simulink model "CascadePID_sim_v2"  (R2024b)
settings: Solver=ode1  StartTime=0.0  StopTime=1  FixedStep=0.005  RelTol=1e-3
undefined symbols (not defined in the file or in its folder): A, b_moment, g, k_thrust, l, M, m, T
libraries: simulink_extras x7, slpidlib x6
settings Model: Creator=Admin  LastModifiedBy=Admin

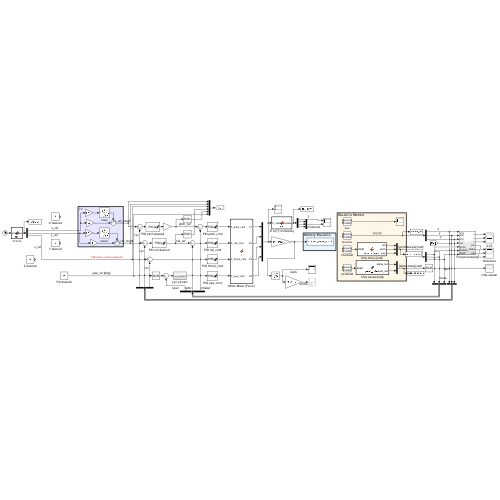
[thumbnail: Simulink's stored preview of the top-level diagram]
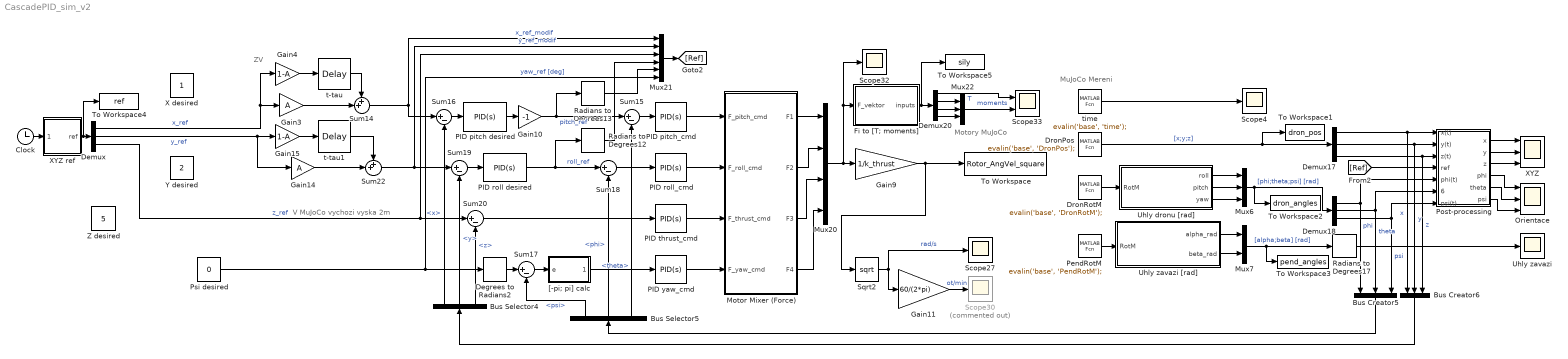
== system CascadePID_sim_v2 ==
  note: Motory MuJoCo
  note: V MuJoCo vychozi vyska 2m
  note: MuJoCo Mereni
  note: ZV
  Bus Creator5 : BusCreator  Inputs=3
  Bus Creator6 : BusCreator  Inputs=3
  Bus Selector4 : BusSelector  OutputSignals=x,y,z
  Bus Selector5 : BusSelector  OutputSignals=psi,phi,theta
  Clock : Clock
  Degrees to Radians2 : simulink_extras/Transformations/Degrees to Radians
  Demux : Demux  Outputs=3
  Demux17 : Demux  Outputs=3
  Demux18 : Demux  Outputs=3
  Demux20 : Demux
  DronPos : MATLABFcn  MATLABFcn=evalin('base', 'DronPos');  OutputDimensions=[3,1]  Output1D=off
  DronRotM : MATLABFcn  MATLABFcn=evalin('base', 'DronRotM');  OutputDimensions=[3,3]  Output1D=off
  Fi to [T; moments] : MATLAB Function  TreatAsAtomicUnit=on
  Gain10 : Gain  Gain=-1
  Gain11 : Gain  Gain=60/(2*pi)
  Gain14 : Gain  Gain=A
  Gain15 : Gain  Gain=1-A
  Gain3 : Gain  Gain=A
  Gain4 : Gain  Gain=1-A
  Gain9 : Gain  Gain=1/k_thrust
  Motor Mixer (Force) : MATLAB Function  TreatAsAtomicUnit=on
  Mux20 : Mux
  Mux21 : Mux  Inputs=6
  Mux22 : Mux  Inputs=3
  Mux6 : Mux  Inputs=3
  Mux7 : Mux  Inputs=2
  Orientace : Scope  NumInputPorts=3
  PID pitch desired : slpidlib/PID Controller  Controller=PID  Form=Parallel  TimeDomain=Continuous-time  UseExternalTs=off  SampleTime=-1  IntegratorMethod=Forward Euler  FilterMethod=Forward Euler  ControllerParametersSource=internal  P=-0.0958604126455568  I=-0.00355407713511052  UseKiTs=off  D=-0.176236133491369  UseExternalDerivativeSource=off  N=18.7292151918558  UseFilter=on  TunerSelectOption=Transfer Function Based (PID Tuner App)  InitialConditionSource=internal  InitialConditionForIntegrator=0  InitialConditionForFilter=0  DifferentiatorICPrevScaledInput=0  ExternalReset=none  TrackingMode=off  Kt=1  LimitOutput=on  SatLimitsSource=internal  UpperSaturationLimit=45*pi/180  LowerSaturationLimit=-45*pi/180  LinearizeAsGain=on  AntiWindupMode=clamping  Kb=1  LimitIntegrator=off  UpperIntegratorSaturationLimit=inf  LowerIntegratorSaturationLimit=-inf  POutMin=[]  POutMax=[]  IOutMin=[]  IOutMax=[]  DOutMin=[]  DOutMax=[]  NOutMin=[]  NOutMax=[]  SumOutMin=[]  SumOutMax=[]  SaturationOutMin=[]  SaturationOutMax=[]  PParamMin=[]  PParamMax=[]  IParamMin=[]  IParamMax=[]  DParamMin=[]  DParamMax=[]  NParamMin=[]  NParamMax=[]  KbParamMin=[]  KbParamMax=[]  KtParamMin=[]  KtParamMax=[]  KbOutMin=[]  KbOutMax=[]  KtOutMin=[]  KtOutMax=[]  IntegratorOutMin=[]  IntegratorOutMax=[]  FilterOutMin=[]  FilterOutMax=[]  SumI1OutMin=[]  SumI1OutMax=[]  SumI2OutMin=[]  SumI2OutMax=[]  SumI3OutMin=[]  SumI3OutMax=[]  SumI4OutMin=[]  SumI4OutMax=[]  SumDOutMin=[]  SumDOutMax=[]  DifferentiatorOutMin=[]  DifferentiatorOutMax=[]  FilterDiffOutCoefMin=[]  FilterDiffOutCoefMax=[]  ReciprocalOutMin=[]  ReciprocalOutMax=[]  SumDenOutMin=[]  SumDenOutMax=[]  SumNumOutMin=[]  SumNumOutMax=[]  DivideOutMin=[]  DivideOutMax=[]  UdiffTsProdOutMin=[]  UdiffTsProdOutMax=[]  NTsProdOutMin=[]  NTsProdOutMax=[]  UintegralTsProdOutMin=[]  UintegralTsProdOutMax=[]  UngainTsProdOutMin=[]  UngainTsProdOutMax=[]  ClampingZeroOutDataTypeStr=Inherit: Inherit via back propagation  ClampingZeroOutMin=[]  ClampingZeroOutMax=[]  FilterDenConstantOutDataTypeStr=Inherit: Inherit via back propagation  FilterDenConstantOutMin=[]  FilterDenConstantOutMax=[]  PCopyOutDataTypeStr=Inherit: Inherit via back propagation  PCopyOutMin=[]  PCopyOutMax=[]  NCopyOutDataTypeStr=Inherit: Inherit via back propagation  NCopyOutMin=[]  NCopyOutMax=[]  IntegratorContinuousStateAttributes=''  IntegratorStateMustResolveToSignalObject=off  IntegratorRTWStateStorageClass=Auto  FilterContinuousStateAttributes=''  FilterStateMustResolveToSignalObject=off  FilterRTWStateStorageClass=Auto  ParallelPVariant=InternalParameters  IdealPVariant=Disabled  IVariant=InternalParameters  DVariant=InternalParameters  IntegratorVariant=Continuous  SatVariant=Enabled  AWVariant=ContClampingParallel  PCopyVariant=Disabled  TRVariant=Disabled  FdbkBlocksVariant=Forward  IdealPFdbkVariant=Disabled  SatFdbkVariant=Disabled  DerivativeFilterVariant=ContFilter  NVariant=InternalParameters  NCopyVariant=Disabled  FilterICVariant=InternalICsFilter  IntegratorICVariant=InternalICs  ExternalResetVariant=Disabled  TRSumVariant=Passthrough  SumFdbkVariant=Disabled  SumVariant=Sum_PID  TsampFilterVariant=InternalTs  TsampNgainVariant=Passthrough  TsampIntegralVariant=Disabled_SignalSpec  ExternalSaturationOutDataTypeStr=Inherit: Same as second input  DerivativeSourceVariant=ErrorSignal  PreIntVariant=InternalPreInt
  PID pitch_cmd : slpidlib/PID Controller  Controller=PID  Form=Parallel  TimeDomain=Continuous-time  UseExternalTs=off  SampleTime=-1  IntegratorMethod=Forward Euler  FilterMethod=Forward Euler  ControllerParametersSource=internal  P=4.88741871339799  I=7.0680919275256  UseKiTs=off  D=0.665907466371152  UseExternalDerivativeSource=off  N=70.3527150062246  UseFilter=on  TunerSelectOption=Transfer Function Based (PID Tuner App)  InitialConditionSource=internal  InitialConditionForIntegrator=0  InitialConditionForFilter=0  DifferentiatorICPrevScaledInput=0  ExternalReset=none  TrackingMode=off  Kt=1  LimitOutput=on  SatLimitsSource=internal  UpperSaturationLimit=0.8  LowerSaturationLimit=-0.8  LinearizeAsGain=off  AntiWindupMode=none  Kb=1  LimitIntegrator=off  UpperIntegratorSaturationLimit=inf  LowerIntegratorSaturationLimit=-inf  POutMin=[]  POutMax=[]  IOutMin=[]  IOutMax=[]  DOutMin=[]  DOutMax=[]  NOutMin=[]  NOutMax=[]  SumOutMin=[]  SumOutMax=[]  SaturationOutMin=[]  SaturationOutMax=[]  PParamMin=[]  PParamMax=[]  IParamMin=[]  IParamMax=[]  DParamMin=[]  DParamMax=[]  NParamMin=[]  NParamMax=[]  KbParamMin=[]  KbParamMax=[]  KtParamMin=[]  KtParamMax=[]  KbOutMin=[]  KbOutMax=[]  KtOutMin=[]  KtOutMax=[]  IntegratorOutMin=[]  IntegratorOutMax=[]  FilterOutMin=[]  FilterOutMax=[]  SumI1OutMin=[]  SumI1OutMax=[]  SumI2OutMin=[]  SumI2OutMax=[]  SumI3OutMin=[]  SumI3OutMax=[]  SumI4OutMin=[]  SumI4OutMax=[]  SumDOutMin=[]  SumDOutMax=[]  DifferentiatorOutMin=[]  DifferentiatorOutMax=[]  FilterDiffOutCoefMin=[]  FilterDiffOutCoefMax=[]  ReciprocalOutMin=[]  ReciprocalOutMax=[]  SumDenOutMin=[]  SumDenOutMax=[]  SumNumOutMin=[]  SumNumOutMax=[]  DivideOutMin=[]  DivideOutMax=[]  UdiffTsProdOutMin=[]  UdiffTsProdOutMax=[]  NTsProdOutMin=[]  NTsProdOutMax=[]  UintegralTsProdOutMin=[]  UintegralTsProdOutMax=[]  UngainTsProdOutMin=[]  UngainTsProdOutMax=[]  ClampingZeroOutDataTypeStr=Inherit: Inherit via back propagation  ClampingZeroOutMin=[]  ClampingZeroOutMax=[]  FilterDenConstantOutDataTypeStr=Inherit: Inherit via back propagation  FilterDenConstantOutMin=[]  FilterDenConstantOutMax=[]  PCopyOutDataTypeStr=Inherit: Inherit via back propagation  PCopyOutMin=[]  PCopyOutMax=[]  NCopyOutDataTypeStr=Inherit: Inherit via back propagation  NCopyOutMin=[]  NCopyOutMax=[]  IntegratorContinuousStateAttributes=''  IntegratorStateMustResolveToSignalObject=off  IntegratorRTWStateStorageClass=Auto  FilterContinuousStateAttributes=''  FilterStateMustResolveToSignalObject=off  FilterRTWStateStorageClass=Auto  ParallelPVariant=InternalParameters  IdealPVariant=Disabled  IVariant=InternalParameters  DVariant=InternalParameters  IntegratorVariant=Continuous  SatVariant=Enabled  AWVariant=Passthrough  PCopyVariant=Disabled  TRVariant=Disabled  FdbkBlocksVariant=Forward  IdealPFdbkVariant=Disabled  SatFdbkVariant=Disabled  DerivativeFilterVariant=ContFilter  NVariant=InternalParameters  NCopyVariant=Disabled  FilterICVariant=InternalICsFilter  IntegratorICVariant=InternalICs  ExternalResetVariant=Disabled  TRSumVariant=Passthrough  SumFdbkVariant=Disabled  SumVariant=Sum_PID  TsampFilterVariant=InternalTs  TsampNgainVariant=Passthrough  TsampIntegralVariant=Disabled_SignalSpec  ExternalSaturationOutDataTypeStr=Inherit: Same as second input  DerivativeSourceVariant=ErrorSignal  PreIntVariant=InternalPreInt
  PID roll desired : slpidlib/PID Controller  Controller=PID  Form=Parallel  TimeDomain=Continuous-time  UseExternalTs=off  SampleTime=-1  IntegratorMethod=Forward Euler  FilterMethod=Forward Euler  ControllerParametersSource=internal  P=-0.0958604126455568  I=-0.00355407713511052  UseKiTs=off  D=-0.176236133491369  UseExternalDerivativeSource=off  N=18.7292151918558  UseFilter=on  TunerSelectOption=Transfer Function Based (PID Tuner App)  InitialConditionSource=internal  InitialConditionForIntegrator=0  InitialConditionForFilter=0  DifferentiatorICPrevScaledInput=0  ExternalReset=none  TrackingMode=off  Kt=1  LimitOutput=on  SatLimitsSource=internal  UpperSaturationLimit=45*pi/180  LowerSaturationLimit=-45*pi/180  LinearizeAsGain=on  AntiWindupMode=clamping  Kb=1  LimitIntegrator=off  UpperIntegratorSaturationLimit=inf  LowerIntegratorSaturationLimit=-inf  POutMin=[]  POutMax=[]  IOutMin=[]  IOutMax=[]  DOutMin=[]  DOutMax=[]  NOutMin=[]  NOutMax=[]  SumOutMin=[]  SumOutMax=[]  SaturationOutMin=[]  SaturationOutMax=[]  PParamMin=[]  PParamMax=[]  IParamMin=[]  IParamMax=[]  DParamMin=[]  DParamMax=[]  NParamMin=[]  NParamMax=[]  KbParamMin=[]  KbParamMax=[]  KtParamMin=[]  KtParamMax=[]  KbOutMin=[]  KbOutMax=[]  KtOutMin=[]  KtOutMax=[]  IntegratorOutMin=[]  IntegratorOutMax=[]  FilterOutMin=[]  FilterOutMax=[]  SumI1OutMin=[]  SumI1OutMax=[]  SumI2OutMin=[]  SumI2OutMax=[]  SumI3OutMin=[]  SumI3OutMax=[]  SumI4OutMin=[]  SumI4OutMax=[]  SumDOutMin=[]  SumDOutMax=[]  DifferentiatorOutMin=[]  DifferentiatorOutMax=[]  FilterDiffOutCoefMin=[]  FilterDiffOutCoefMax=[]  ReciprocalOutMin=[]  ReciprocalOutMax=[]  SumDenOutMin=[]  SumDenOutMax=[]  SumNumOutMin=[]  SumNumOutMax=[]  DivideOutMin=[]  DivideOutMax=[]  UdiffTsProdOutMin=[]  UdiffTsProdOutMax=[]  NTsProdOutMin=[]  NTsProdOutMax=[]  UintegralTsProdOutMin=[]  UintegralTsProdOutMax=[]  UngainTsProdOutMin=[]  UngainTsProdOutMax=[]  ClampingZeroOutDataTypeStr=Inherit: Inherit via back propagation  ClampingZeroOutMin=[]  ClampingZeroOutMax=[]  FilterDenConstantOutDataTypeStr=Inherit: Inherit via back propagation  FilterDenConstantOutMin=[]  FilterDenConstantOutMax=[]  PCopyOutDataTypeStr=Inherit: Inherit via back propagation  PCopyOutMin=[]  PCopyOutMax=[]  NCopyOutDataTypeStr=Inherit: Inherit via back propagation  NCopyOutMin=[]  NCopyOutMax=[]  IntegratorContinuousStateAttributes=''  IntegratorStateMustResolveToSignalObject=off  IntegratorRTWStateStorageClass=Auto  FilterContinuousStateAttributes=''  FilterStateMustResolveToSignalObject=off  FilterRTWStateStorageClass=Auto  ParallelPVariant=InternalParameters  IdealPVariant=Disabled  IVariant=InternalParameters  DVariant=InternalParameters  IntegratorVariant=Continuous  SatVariant=Enabled  AWVariant=ContClampingParallel  PCopyVariant=Disabled  TRVariant=Disabled  FdbkBlocksVariant=Forward  IdealPFdbkVariant=Disabled  SatFdbkVariant=Disabled  DerivativeFilterVariant=ContFilter  NVariant=InternalParameters  NCopyVariant=Disabled  FilterICVariant=InternalICsFilter  IntegratorICVariant=InternalICs  ExternalResetVariant=Disabled  TRSumVariant=Passthrough  SumFdbkVariant=Disabled  SumVariant=Sum_PID  TsampFilterVariant=InternalTs  TsampNgainVariant=Passthrough  TsampIntegralVariant=Disabled_SignalSpec  ExternalSaturationOutDataTypeStr=Inherit: Same as second input  DerivativeSourceVariant=ErrorSignal  PreIntVariant=InternalPreInt
  PID roll_cmd : slpidlib/PID Controller  Controller=PID  Form=Parallel  TimeDomain=Continuous-time  UseExternalTs=off  SampleTime=-1  IntegratorMethod=Forward Euler  FilterMethod=Forward Euler  ControllerParametersSource=internal  P=4.88741871339799  I=7.0680919275256  UseKiTs=off  D=0.665907466371152  UseExternalDerivativeSource=off  N=70.3527150062246  UseFilter=on  TunerSelectOption=Transfer Function Based (PID Tuner App)  InitialConditionSource=internal  InitialConditionForIntegrator=0  InitialConditionForFilter=0  DifferentiatorICPrevScaledInput=0  ExternalReset=none  TrackingMode=off  Kt=1  LimitOutput=on  SatLimitsSource=internal  UpperSaturationLimit=0.8  LowerSaturationLimit=-0.8  LinearizeAsGain=off  AntiWindupMode=none  Kb=1  LimitIntegrator=off  UpperIntegratorSaturationLimit=inf  LowerIntegratorSaturationLimit=-inf  POutMin=[]  POutMax=[]  IOutMin=[]  IOutMax=[]  DOutMin=[]  DOutMax=[]  NOutMin=[]  NOutMax=[]  SumOutMin=[]  SumOutMax=[]  SaturationOutMin=[]  SaturationOutMax=[]  PParamMin=[]  PParamMax=[]  IParamMin=[]  IParamMax=[]  DParamMin=[]  DParamMax=[]  NParamMin=[]  NParamMax=[]  KbParamMin=[]  KbParamMax=[]  KtParamMin=[]  KtParamMax=[]  KbOutMin=[]  KbOutMax=[]  KtOutMin=[]  KtOutMax=[]  IntegratorOutMin=[]  IntegratorOutMax=[]  FilterOutMin=[]  FilterOutMax=[]  SumI1OutMin=[]  SumI1OutMax=[]  SumI2OutMin=[]  SumI2OutMax=[]  SumI3OutMin=[]  SumI3OutMax=[]  SumI4OutMin=[]  SumI4OutMax=[]  SumDOutMin=[]  SumDOutMax=[]  DifferentiatorOutMin=[]  DifferentiatorOutMax=[]  FilterDiffOutCoefMin=[]  FilterDiffOutCoefMax=[]  ReciprocalOutMin=[]  ReciprocalOutMax=[]  SumDenOutMin=[]  SumDenOutMax=[]  SumNumOutMin=[]  SumNumOutMax=[]  DivideOutMin=[]  DivideOutMax=[]  UdiffTsProdOutMin=[]  UdiffTsProdOutMax=[]  NTsProdOutMin=[]  NTsProdOutMax=[]  UintegralTsProdOutMin=[]  UintegralTsProdOutMax=[]  UngainTsProdOutMin=[]  UngainTsProdOutMax=[]  ClampingZeroOutDataTypeStr=Inherit: Inherit via back propagation  ClampingZeroOutMin=[]  ClampingZeroOutMax=[]  FilterDenConstantOutDataTypeStr=Inherit: Inherit via back propagation  FilterDenConstantOutMin=[]  FilterDenConstantOutMax=[]  PCopyOutDataTypeStr=Inherit: Inherit via back propagation  PCopyOutMin=[]  PCopyOutMax=[]  NCopyOutDataTypeStr=Inherit: Inherit via back propagation  NCopyOutMin=[]  NCopyOutMax=[]  IntegratorContinuousStateAttributes=''  IntegratorStateMustResolveToSignalObject=off  IntegratorRTWStateStorageClass=Auto  FilterContinuousStateAttributes=''  FilterStateMustResolveToSignalObject=off  FilterRTWStateStorageClass=Auto  ParallelPVariant=InternalParameters  IdealPVariant=Disabled  IVariant=InternalParameters  DVariant=InternalParameters  IntegratorVariant=Continuous  SatVariant=Enabled  AWVariant=Passthrough  PCopyVariant=Disabled  TRVariant=Disabled  FdbkBlocksVariant=Forward  IdealPFdbkVariant=Disabled  SatFdbkVariant=Disabled  DerivativeFilterVariant=ContFilter  NVariant=InternalParameters  NCopyVariant=Disabled  FilterICVariant=InternalICsFilter  IntegratorICVariant=InternalICs  ExternalResetVariant=Disabled  TRSumVariant=Passthrough  SumFdbkVariant=Disabled  SumVariant=Sum_PID  TsampFilterVariant=InternalTs  TsampNgainVariant=Passthrough  TsampIntegralVariant=Disabled_SignalSpec  ExternalSaturationOutDataTypeStr=Inherit: Same as second input  DerivativeSourceVariant=ErrorSignal  PreIntVariant=InternalPreInt
  PID thrust_cmd : slpidlib/PID Controller  Controller=PID  Form=Parallel  TimeDomain=Continuous-time  UseExternalTs=off  SampleTime=-1  IntegratorMethod=Forward Euler  FilterMethod=Forward Euler  ControllerParametersSource=internal  P=3.2536  I=0.7965  UseKiTs=off  D=3.0648  UseExternalDerivativeSource=off  N=11.4924  UseFilter=on  TunerSelectOption=Transfer Function Based (PID Tuner App)  InitialConditionSource=internal  InitialConditionForIntegrator=(M+m)*g/4  InitialConditionForFilter=2.05  DifferentiatorICPrevScaledInput=0  ExternalReset=none  TrackingMode=off  Kt=1  LimitOutput=on  SatLimitsSource=internal  UpperSaturationLimit=34.3  LowerSaturationLimit=2.05  LinearizeAsGain=off  AntiWindupMode=clamping  Kb=1  LimitIntegrator=off  UpperIntegratorSaturationLimit=inf  LowerIntegratorSaturationLimit=-inf  POutMin=[]  POutMax=[]  IOutMin=[]  IOutMax=[]  DOutMin=[]  DOutMax=[]  NOutMin=[]  NOutMax=[]  SumOutMin=[]  SumOutMax=[]  SaturationOutMin=[]  SaturationOutMax=[]  PParamMin=[]  PParamMax=[]  IParamMin=[]  IParamMax=[]  DParamMin=[]  DParamMax=[]  NParamMin=[]  NParamMax=[]  KbParamMin=[]  KbParamMax=[]  KtParamMin=[]  KtParamMax=[]  KbOutMin=[]  KbOutMax=[]  KtOutMin=[]  KtOutMax=[]  IntegratorOutMin=[]  IntegratorOutMax=[]  FilterOutMin=[]  FilterOutMax=[]  SumI1OutMin=[]  SumI1OutMax=[]  SumI2OutMin=[]  SumI2OutMax=[]  SumI3OutMin=[]  SumI3OutMax=[]  SumI4OutMin=[]  SumI4OutMax=[]  SumDOutMin=[]  SumDOutMax=[]  DifferentiatorOutMin=[]  DifferentiatorOutMax=[]  FilterDiffOutCoefMin=[]  FilterDiffOutCoefMax=[]  ReciprocalOutMin=[]  ReciprocalOutMax=[]  SumDenOutMin=[]  SumDenOutMax=[]  SumNumOutMin=[]  SumNumOutMax=[]  DivideOutMin=[]  DivideOutMax=[]  UdiffTsProdOutMin=[]  UdiffTsProdOutMax=[]  NTsProdOutMin=[]  NTsProdOutMax=[]  UintegralTsProdOutMin=[]  UintegralTsProdOutMax=[]  UngainTsProdOutMin=[]  UngainTsProdOutMax=[]  ClampingZeroOutDataTypeStr=Inherit: Inherit via back propagation  ClampingZeroOutMin=[]  ClampingZeroOutMax=[]  FilterDenConstantOutDataTypeStr=Inherit: Inherit via back propagation  FilterDenConstantOutMin=[]  FilterDenConstantOutMax=[]  PCopyOutDataTypeStr=Inherit: Inherit via back propagation  PCopyOutMin=[]  PCopyOutMax=[]  NCopyOutDataTypeStr=Inherit: Inherit via back propagation  NCopyOutMin=[]  NCopyOutMax=[]  IntegratorContinuousStateAttributes=''  IntegratorStateMustResolveToSignalObject=off  IntegratorRTWStateStorageClass=Auto  FilterContinuousStateAttributes=''  FilterStateMustResolveToSignalObject=off  FilterRTWStateStorageClass=Auto  ParallelPVariant=InternalParameters  IdealPVariant=Disabled  IVariant=InternalParameters  DVariant=InternalParameters  IntegratorVariant=Continuous  SatVariant=Enabled  AWVariant=ContClampingParallel  PCopyVariant=Disabled  TRVariant=Disabled  FdbkBlocksVariant=Forward  IdealPFdbkVariant=Disabled  SatFdbkVariant=Disabled  DerivativeFilterVariant=ContFilter  NVariant=InternalParameters  NCopyVariant=Disabled  FilterICVariant=InternalICsFilter  IntegratorICVariant=InternalICs  ExternalResetVariant=Disabled  TRSumVariant=Passthrough  SumFdbkVariant=Disabled  SumVariant=Sum_PID  TsampFilterVariant=InternalTs  TsampNgainVariant=Passthrough  TsampIntegralVariant=Disabled_SignalSpec  ExternalSaturationOutDataTypeStr=Inherit: Same as second input  DerivativeSourceVariant=ErrorSignal  PreIntVariant=InternalPreInt
  PID yaw_cmd : slpidlib/PID Controller  Controller=PID  Form=Parallel  TimeDomain=Continuous-time  UseExternalTs=off  SampleTime=-1  IntegratorMethod=Forward Euler  FilterMethod=Forward Euler  ControllerParametersSource=internal  P=1.76936488001119  I=0.499479618576994  UseKiTs=off  D=1.26710500363477  UseExternalDerivativeSource=off  N=13.1063871491015  UseFilter=on  TunerSelectOption=Transfer Function Based (PID Tuner App)  InitialConditionSource=internal  InitialConditionForIntegrator=0  InitialConditionForFilter=0  DifferentiatorICPrevScaledInput=0  ExternalReset=none  TrackingMode=off  Kt=1  LimitOutput=on  SatLimitsSource=internal  UpperSaturationLimit=0.4  LowerSaturationLimit=-0.4  LinearizeAsGain=off  AntiWindupMode=clamping  Kb=1  LimitIntegrator=off  UpperIntegratorSaturationLimit=inf  LowerIntegratorSaturationLimit=-inf  POutMin=[]  POutMax=[]  IOutMin=[]  IOutMax=[]  DOutMin=[]  DOutMax=[]  NOutMin=[]  NOutMax=[]  SumOutMin=[]  SumOutMax=[]  SaturationOutMin=[]  SaturationOutMax=[]  PParamMin=[]  PParamMax=[]  IParamMin=[]  IParamMax=[]  DParamMin=[]  DParamMax=[]  NParamMin=[]  NParamMax=[]  KbParamMin=[]  KbParamMax=[]  KtParamMin=[]  KtParamMax=[]  KbOutMin=[]  KbOutMax=[]  KtOutMin=[]  KtOutMax=[]  IntegratorOutMin=[]  IntegratorOutMax=[]  FilterOutMin=[]  FilterOutMax=[]  SumI1OutMin=[]  SumI1OutMax=[]  SumI2OutMin=[]  SumI2OutMax=[]  SumI3OutMin=[]  SumI3OutMax=[]  SumI4OutMin=[]  SumI4OutMax=[]  SumDOutMin=[]  SumDOutMax=[]  DifferentiatorOutMin=[]  DifferentiatorOutMax=[]  FilterDiffOutCoefMin=[]  FilterDiffOutCoefMax=[]  ReciprocalOutMin=[]  ReciprocalOutMax=[]  SumDenOutMin=[]  SumDenOutMax=[]  SumNumOutMin=[]  SumNumOutMax=[]  DivideOutMin=[]  DivideOutMax=[]  UdiffTsProdOutMin=[]  UdiffTsProdOutMax=[]  NTsProdOutMin=[]  NTsProdOutMax=[]  UintegralTsProdOutMin=[]  UintegralTsProdOutMax=[]  UngainTsProdOutMin=[]  UngainTsProdOutMax=[]  ClampingZeroOutDataTypeStr=Inherit: Inherit via back propagation  ClampingZeroOutMin=[]  ClampingZeroOutMax=[]  FilterDenConstantOutDataTypeStr=Inherit: Inherit via back propagation  FilterDenConstantOutMin=[]  FilterDenConstantOutMax=[]  PCopyOutDataTypeStr=Inherit: Inherit via back propagation  PCopyOutMin=[]  PCopyOutMax=[]  NCopyOutDataTypeStr=Inherit: Inherit via back propagation  NCopyOutMin=[]  NCopyOutMax=[]  IntegratorContinuousStateAttributes=''  IntegratorStateMustResolveToSignalObject=off  IntegratorRTWStateStorageClass=Auto  FilterContinuousStateAttributes=''  FilterStateMustResolveToSignalObject=off  FilterRTWStateStorageClass=Auto  ParallelPVariant=InternalParameters  IdealPVariant=Disabled  IVariant=InternalParameters  DVariant=InternalParameters  IntegratorVariant=Continuous  SatVariant=Enabled  AWVariant=ContClampingParallel  PCopyVariant=Disabled  TRVariant=Disabled  FdbkBlocksVariant=Forward  IdealPFdbkVariant=Disabled  SatFdbkVariant=Disabled  DerivativeFilterVariant=ContFilter  NVariant=InternalParameters  NCopyVariant=Disabled  FilterICVariant=InternalICsFilter  IntegratorICVariant=InternalICs  ExternalResetVariant=Disabled  TRSumVariant=Passthrough  SumFdbkVariant=Disabled  SumVariant=Sum_PID  TsampFilterVariant=InternalTs  TsampNgainVariant=Passthrough  TsampIntegralVariant=Disabled_SignalSpec  ExternalSaturationOutDataTypeStr=Inherit: Same as second input  DerivativeSourceVariant=ErrorSignal  PreIntVariant=InternalPreInt
  PendRotM : MATLABFcn  MATLABFcn=evalin('base', 'PendRotM');  OutputDimensions=[3,3]  Output1D=off
  Post-processing : Subsystem
  Psi desired : Constant  Value=0
  Radians to Degrees12 : simulink_extras/Transformations/Radians to Degrees
  Radians to Degrees13 : simulink_extras/Transformations/Radians to Degrees
  Radians to Degrees17 : simulink_extras/Transformations/Radians to Degrees
  Scope27 : Scope
  Scope30 : Scope  Commented=on
  Scope32 : Scope
  Scope33 : Scope  NumInputPorts=2
  Scope4 : Scope
  Sqrt2 : Sqrt
  Sum14 : Sum  Inputs=++|
  Sum{15..20} (6 alike) : Sum  Inputs=|+-
  Sum22 : Sum  Inputs=++|
  To Workspace : ToWorkspace  VariableName=Rotor_AngVel_square  SampleTime=-1
  To Workspace1 : ToWorkspace  VariableName=dron_pos  SaveFormat=Timeseries  SampleTime=-1
  To Workspace2 : ToWorkspace  VariableName=dron_angles  SaveFormat=Timeseries  SampleTime=-1
  To Workspace3 : ToWorkspace  VariableName=pend_angles  SaveFormat=Timeseries  SampleTime=-1
  To Workspace4 : ToWorkspace  VariableName=ref  SaveFormat=Timeseries  SampleTime=-1
  To Workspace5 : ToWorkspace  VariableName=sily  SaveFormat=Timeseries  SampleTime=-1
  Uhly dronu [rad] : MATLAB Function  TreatAsAtomicUnit=on
  Uhly zavazi : Scope
  Uhly zavazi [rad] : MATLAB Function  TreatAsAtomicUnit=on
  X desired : Constant
  XYZ : Scope  NumInputPorts=3
  XYZ ref : MATLAB Function  TreatAsAtomicUnit=on
  Y desired : Constant  Value=2
  Z desired : Constant  Value=5
  "[-pi; pi] calc" : Subsystem
  t-tau : TransportDelay  DelayTime=T
  t-tau1 : TransportDelay  DelayTime=T
  time : MATLABFcn  MATLABFcn=evalin('base', 'time');  Output1D=off
  wires:
  Clock/1 -> XYZ ref/1(simtime)
  DronPos/1 -> Demux17/1, To Workspace1/1  "[x;y;z]"
  Mux6/1 -> Demux18/1, To Workspace2/1  "[phi;theta;psi] [rad]"
  Mux7/1 -> To Workspace3/1, Radians to Degrees17/1  "[alpha;beta] [rad]"
  DronRotM/1 -> Uhly dronu [rad]/1(RotM)
  Uhly dronu [rad]/2(pitch) -> Mux6/2
  Uhly zavazi [rad]/2(beta_rad) -> Mux7/2
  Uhly dronu [rad]/3(yaw) -> Mux6/3
  PendRotM/1 -> Uhly zavazi [rad]/1(RotM)
  Uhly dronu [rad]/1(roll) -> Mux6/1
  Uhly zavazi [rad]/1(alpha_rad) -> Mux7/1
  time/1 -> Scope4/1
  Demux20/2 -> Mux22/1
  Radians to Degrees13/1 -> Mux21/5
  PID thrust_cmd/1 -> Motor Mixer (Force)/3(F_thrust_cmd)
  Gain15/1 -> t-tau1/1
  Radians to Degrees17/1 -> Uhly zavazi/1
  Demux20/1 -> Scope33/1  "T"
  Post-processing/5(theta) -> Orientace/2
  Post-processing/3(z) -> XYZ/3
  Sum22/1 -> Mux21/2, Sum19/1  "y_ref_modif"
  Sum18/1 -> PID roll_cmd/1
  Demux18/3 -> Post-processing/7(psi(t)), Bus Creator5/3  "psi"
  Demux18/1 -> Post-processing/5(phi(t)), Bus Creator5/1  "phi"
  Post-processing/1(x) -> XYZ/1
  Sum17/1 -> "[-pi; pi] calc"/1(e)
  Gain4/1 -> t-tau/1
  Bus Selector4/3 -> Sum20/2  "<z>"
  Psi desired/1 -> Mux21/6, Degrees to Radians2/1  "yaw_ref [deg]"
  PID roll_cmd/1 -> Motor Mixer (Force)/2(F_roll_cmd)
  PID roll desired/1 -> Sum18/1, Radians to Degrees12/1  "roll_ref"
  "[-pi; pi] calc"/1(e_norm) -> PID yaw_cmd/1
  Motor Mixer (Force)/1(F1) -> Mux20/1
  Demux/1 -> Gain4/1, Gain3/1  "x_ref"
  Bus Selector4/1 -> Sum16/2  "<x>"
  Gain11/1 -> Scope30/1  "ot/min"
  Gain3/1 -> Sum14/2
  PID pitch_cmd/1 -> Motor Mixer (Force)/1(F_pitch_cmd)
  Demux20/3 -> Mux22/2
  Bus Selector5/2 -> Sum18/2  "<phi>"
  Demux18/2 -> Post-processing/6(theta(t)), Bus Creator5/2  "theta"
  Bus Selector4/2 -> Sum19/2  "<y>"
  Bus Selector5/1 -> Sum17/2  "<psi>"
  Degrees to Radians2/1 -> Sum17/1
  Demux/3 -> Mux21/3, Sum20/1  "z_ref"
  Motor Mixer (Force)/3(F3) -> Mux20/3
  [Ref] -> Post-processing/4(ref)
  Post-processing/2(y) -> XYZ/2
  Demux17/3 -> Post-processing/3(z(t)), Bus Creator6/3  "z"
  Sum20/1 -> PID thrust_cmd/1
  Mux22/1 -> Scope33/2  "moments"
  Gain14/1 -> Sum22/2
  Sum14/1 -> Sum16/1, Mux21/1  "x_ref_modif"
  t-tau1/1 -> Sum22/1
  Bus Creator6/1 -> Bus Selector4/1
  Mux20/1 -> Scope32/1, Fi to [T; moments]/1(F_vektor), Gain9/1
  Sum15/1 -> PID pitch_cmd/1
  Sum19/1 -> PID roll desired/1
  Gain10/1 -> Sum15/1, Radians to Degrees13/1  "pitch_ref"
  PID pitch desired/1 -> Gain10/1
  Sqrt2/1 -> Gain11/1, Scope27/1  "rad/s"
  Demux17/1 -> Post-processing/1(x(t)), Bus Creator6/1  "x"
  Motor Mixer (Force)/2(F2) -> Mux20/2
  Demux/2 -> Gain14/1, Gain15/1  "y_ref"
  Fi to [T; moments]/1(inputs) -> To Workspace5/1, Demux20/1
  Bus Creator5/1 -> Bus Selector5/1
  Post-processing/6(psi) -> Orientace/3
  Mux21/1 -> [Ref]
  Sum16/1 -> PID pitch desired/1
  Radians to Degrees12/1 -> Mux21/4
  t-tau/1 -> Sum14/1
  Bus Selector5/3 -> Sum15/2  "<theta>"
  Demux20/4 -> Mux22/3
  Demux17/2 -> Post-processing/2(y(t)), Bus Creator6/2  "y"
  PID yaw_cmd/1 -> Motor Mixer (Force)/4(F_yaw_cmd)
  Post-processing/4(phi) -> Orientace/1
  Motor Mixer (Force)/4(F4) -> Mux20/4
  Gain9/1 -> To Workspace/1, Sqrt2/1
  XYZ ref/1(ref) -> To Workspace4/1, Demux/1

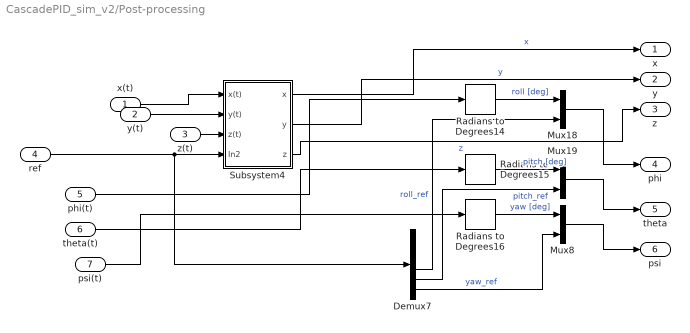
== system CascadePID_sim_v2/Post-processing ==
  x(t) : Inport
  y(t) : Inport  Port=2
  z(t) : Inport  Port=3
  ref : Inport  Port=4
  phi(t) : Inport  Port=5
  theta(t) : Inport  Port=6
  psi(t) : Inport  Port=7
  Demux7 : Demux  Outputs=6
  Mux18 : Mux  Inputs=2
  Mux19 : Mux  Inputs=2
  Mux8 : Mux  Inputs=2
  Radians to Degrees14 : simulink_extras/Transformations/Radians to Degrees
  Radians to Degrees15 : simulink_extras/Transformations/Radians to Degrees
  Radians to Degrees16 : simulink_extras/Transformations/Radians to Degrees
  Subsystem4 : Subsystem
  x : Outport
  y : Outport  Port=2
  z : Outport  Port=3
  phi : Outport  Port=4
  theta : Outport  Port=5
  psi : Outport  Port=6
  wires:
  Radians to Degrees16/1 -> Mux8/1  "yaw [deg]"
  ref/1 -> Subsystem4/4(In2), Demux7/1
  Demux7/6 -> Mux8/2  "yaw_ref"
  theta(t)/1 -> Radians to Degrees15/1
  Demux7/4 -> Mux18/2  "roll_ref"
  Demux7/5 -> Mux19/2  "pitch_ref"
  Mux18/1 -> phi/1
  Subsystem4/3(z) -> z/1  "z"
  Radians to Degrees14/1 -> Mux18/1  "roll [deg]"
  Radians to Degrees15/1 -> Mux19/1  "pitch [deg]"
  Subsystem4/2(y) -> y/1  "y"
  x(t)/1 -> Subsystem4/1(x(t))
  y(t)/1 -> Subsystem4/2(y(t))
  psi(t)/1 -> Radians to Degrees16/1
  phi(t)/1 -> Radians to Degrees14/1
  Subsystem4/1(x) -> x/1  "x"
  Mux8/1 -> psi/1
  z(t)/1 -> Subsystem4/3(z(t))
  Mux19/1 -> theta/1

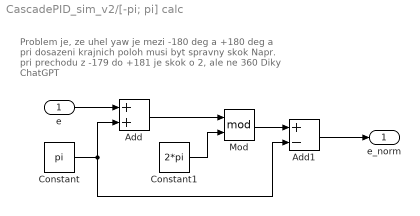
== system CascadePID_sim_v2/[-pi; pi] calc ==
  note: Problem je, ze uhel yaw je mezi -180 deg a +180 deg
      | a pri dosazeni krajnich poloh musi byt spravny skok
      | Napr. pri prechodu z -179 do +181 je skok o 2, ale ne 360
      | Diky ChatGPT
  e : Inport
  Add : Sum
  Add1 : Sum  Inputs=+-
  Constant : Constant  Value=pi
  Constant1 : Constant  Value=2*pi
  Mod : Math  Operator=mod
  e_norm : Outport
  wires:
  e/1 -> Add/1
  Add/1 -> Mod/1
  Constant/1 -> Add1/2, Add/2
  Constant1/1 -> Mod/2
  Mod/1 -> Add1/1
  Add1/1 -> e_norm/1

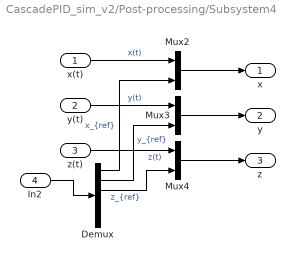
== system CascadePID_sim_v2/Post-processing/Subsystem4 ==
  x(t) : Inport
  y(t) : Inport  Port=2
  z(t) : Inport  Port=3
  In2 : Inport  Port=4
  Demux : Demux  Outputs=6
  Mux2 : Mux  Inputs=2
  Mux3 : Mux  Inputs=2
  Mux4 : Mux  Inputs=2
  x : Outport
  y : Outport  Port=2
  z : Outport  Port=3
  wires:
  Demux/2 -> Mux3/2  "y_{ref}"
  Mux4/1 -> z/1
  y(t)/1 -> Mux3/1  "y(t)"
  Mux3/1 -> y/1
  Demux/1 -> Mux2/2  "x_{ref}"
  Demux/3 -> Mux4/2  "z_{ref}"
  Mux2/1 -> x/1
  In2/1 -> Demux/1
  x(t)/1 -> Mux2/1  "x(t)"
  z(t)/1 -> Mux4/1  "z(t)"

== matlab function CascadePID_sim_v2/Uhly dronu [rad] ==
  data: RotM input; roll output; pitch output; yaw output
function [roll, pitch, yaw] = quad_attitude(RotM)
% matice rotace koptery z Python, vuci svetu!!!
% rotm2eul prevadi na Eulerove uhly
radians = rotm2eul(RotM, 'ZYX'); % pouzivam poradi ZYX

% roll = kolem x, pitch = kolem y, yaw = kolem z
yaw = radians(1);
pitch = radians(2);
roll = radians(3);
end

== matlab function CascadePID_sim_v2/XYZ ref ==
  data: ref output; simtime input
function ref = fcn(simtime)
% pouze poloha, yaw_ref=0
if simtime < 1
    ref = [0;0;2];
elseif simtime < 6
    ref = [3;3;2];
elseif simtime < 10
    ref = [3;3;6];
elseif simtime < 15
    ref = [3;0;6];
elseif simtime < 22
    ref = [3;-3;8];
elseif simtime < 30
    ref = [-3;0;6];
elseif simtime < 35
    ref = [-3;3;6];
elseif simtime < 38
    ref = [-3;3;3];
elseif simtime < 40
    ref = [0;3;2];
elseif simtime < 45 % -> simtime 50s
    ref = [0;0;2];
else
    ref = [0;0;2]; % pokud co, tak pocatecni poloha
end

== matlab function CascadePID_sim_v2/Uhly zavazi [rad] ==
  data: RotM input; alpha_rad output; beta_rad output
function [alpha_rad, beta_rad] = pend_orient(RotM)
% Расчет углов альфа и бета маятника

% Вектор маятника
rope_vector = RotM * [0; 0; -1];

% Расчет угла альфа
rope_vector_xz = rope_vector([1, 3]); % Компоненты x и z
z_axis = [0; -1];
cos_alpha = dot(rope_vector_xz, z_axis) / (norm(rope_vector_xz) * norm(z_axis));
cos_alpha = max(-1, min(1, cos_alpha)); % Ограничиваем в диапазоне [-1, 1]
alpha = acos(cos_alpha);
if rope_vector(1) < 0
    alpha = -alpha;
end

% Расчет угла бета
rope_vector_xz_3 = [rope_vector(1); 0; rope_vector(3)];
cos_beta = dot(rope_vector, rope_vector_xz_3) / (norm(rope_vector) * norm(rope_vector_xz_3));
cos_beta = max(-1, min(1, cos_beta)); % Ограничиваем в диапазоне [-1, 1]
beta = acos(cos_beta);
if rope_vector(2) < 0
    beta = -beta;
end

% Округляем до 5 знаков после запятой
% alpha_rad = round(alpha, 5); %[rad]
% beta_rad = round(beta, 5); %[rad]
alpha_rad = alpha;
beta_rad = beta;

== matlab function CascadePID_sim_v2/Fi to [T; moments] ==
  data: F_vektor input; inputs output; k_thrust parameter; b_moment parameter; l parameter
function inputs = fcn(F_vektor, k_thrust, b_moment, l)
% Dle X tvaru kvadrokoptery dopocitavam 
% celkovou tahovou silu T a tri momenty
F1 = F_vektor(1);
F2 = F_vektor(2);
F3 = F_vektor(3);
F4 = F_vektor(4);

T = F1+F2+F3+F4;
Tau_phi = l*(F1+F4-F2-F3);
Tau_theta = l*(F3+F4-F1-F2);
Tau_psi = b_moment/k_thrust*(F1-F2+F3-F4);

inputs = [T; Tau_phi; Tau_theta; Tau_psi];

== matlab function CascadePID_sim_v2/Motor Mixer (Force) ==
  data: F_pitch_cmd input; F_roll_cmd input; F_thrust_cmd input; F1 output; F_yaw_cmd input; F2 output; F3 output; F4 output
function [F1, F2, F3, F4] = fcn(F_pitch_cmd, F_roll_cmd, F_thrust_cmd, F_yaw_cmd)

% _cmd definuji jednotlive tahove sily Ti na motorech
% -> lze jednoduse prepocitat na nutne otacky
F1 = F_thrust_cmd+F_roll_cmd-F_pitch_cmd+F_yaw_cmd; %[N]
F2 = F_thrust_cmd-F_roll_cmd-F_pitch_cmd-F_yaw_cmd;
F3 = F_thrust_cmd-F_roll_cmd+F_pitch_cmd+F_yaw_cmd;
F4 = F_thrust_cmd+F_roll_cmd+F_pitch_cmd-F_yaw_cmd;
